simulink model "p1_digital_twin"  (R2023a)
settings: Solver=FixedStepDiscrete  StartTime=0.0  StopTime=10  FixedStep=Ts  RelTol=1e-3  EnableMultiTasking=on
undefined symbols (not defined in the file or in its folder): ack, cpr_handwheel, cpr_steering, DiscIntNeverNeededParam, hal_filter_den, hal_filter_num, n_drive, n_handwheel, n_steering, p1params, param, sr, steering_limit, Ts, wc
libraries: simulink x7
(part 4 of 4)

== system p1_digital_twin/Driver and Controller Input/Steering Controller/HAL-9000/Chirp Signal ==
  note: freqSlope = deltaFreq/targetTime;
      | instantaneousFreq(t) = freqSlope*t + initialFreq;
      | intantaneousPhase(t) = integral(instFreq) = ...
      |       0.5*freqSlope*t^2 + initialFreq*t;
      | outputSignal(t) = sin(instantaneousPhase(t));
  Start Time : Inport
  Digital Clock : DigitalClock  SampleTime=Ts
  Gain : Gain  DisableCoverage=on  Gain=0.5  OutDataTypeStr=Inherit: Same as input  ParamDataTypeStr=Inherit: Same as input
  Output : Trigonometry
  Product : Product  DisableCoverage=on  Inputs=*/  InputSameDT=on  SaturateOnIntegerOverflow=on  OutDataTypeStr=Inherit: Same as first input
  Product1 : Product  DisableCoverage=on  InputSameDT=on  SaturateOnIntegerOverflow=on  OutDataTypeStr=Inherit: Same as first input
  Product2 : Product  DisableCoverage=on  InputSameDT=on  SaturateOnIntegerOverflow=on  OutDataTypeStr=Inherit: Same as first input
  Saturation : Saturate  UpperLimit=duration  LowerLimit=0
  Sum : Sum  DisableCoverage=on  Inputs=|++  InputSameDT=on  SaturateOnIntegerOverflow=on  OutDataTypeStr=Inherit: Same as first input
  Sum1 : Sum  DisableCoverage=on  Inputs=-+|  InputSameDT=on  SaturateOnIntegerOverflow=on  OutDataTypeStr=Inherit: Same as first input
  deltaFreq : Constant  DisableCoverage=on  Value=2*pi*(f2-f1)
  initialFreq : Constant  DisableCoverage=on  Value=2*pi*f1
  targetTime : Constant  DisableCoverage=on  Value=T
  Out2 : Outport
  wires:
  Sum1/1 -> Saturation/1
  Digital Clock/1 -> Sum1/2
  Start Time/1 -> Sum1/1
  deltaFreq/1 -> Product/1
  targetTime/1 -> Product/2
  Product/1 -> Gain/1
  Gain/1 -> Product1/2
  Product1/1 -> Sum/1
  initialFreq/1 -> Sum/2
  Sum/1 -> Product2/2
  Product2/1 -> Output/1
  Output/1 -> Out2/1
  Saturation/1 -> Product1/1, Product2/1

== system p1_digital_twin/Driver and Controller Input/Steering Controller/HAL-9000/Double chirp ==
  In1 : Inport
  Chirp One : Subsystem  mask(chirp){f1=startfreq, T=duration/2, f2=endfreq, VectorParams1D=on}
      mask prompts: f1 "Initial frequency (Hz):"; T "Target time (secs):"; f2 "Frequency at target time (Hz):"; VectorParams1D "Interpret vectors parameters as 1-D"
      mask help: Output a linear chirp signal (sine wave whose frequency varies linearly with time).
      mask init: same as p1_digital_twin/Driver and Controller Input/Steering Controller/HAL-9000/Chirp Signal
      mask Help: The chirp signal has linearly increasing frequency with time.  This block can be used for spectral analysis of nonlinear systems.
      mask Display: plot(t,sin(t.*t))
  Chirp Two : Subsystem  mask(chirp){f1=startfreq, T=duration/2, f2=endfreq, VectorParams1D=on}
      mask prompts: f1 "Initial frequency (Hz):"; T "Target time (secs):"; f2 "Frequency at target time (Hz):"; VectorParams1D "Interpret vectors parameters as 1-D"
      mask help: Output a linear chirp signal (sine wave whose frequency varies linearly with time).
      mask init: same as p1_digital_twin/Driver and Controller Input/Steering Controller/HAL-9000/Chirp Signal
      mask Help: The chirp signal has linearly increasing frequency with time.  This block can be used for spectral analysis of nonlinear systems.
      mask Display: plot(t,sin(t.*t))
  Digital Clock : DigitalClock  SampleTime=Ts
  Relational Operator : RelationalOperator  Operator=<=  OutDataTypeStr=float('double')  InputSameDT=off
  Sum : Sum  DisableCoverage=on  Inputs=++|  InputSameDT=on  SaturateOnIntegerOverflow=on  OutDataTypeStr=Inherit: Same as first input
  Switch : Switch  Threshold=.5  SaturateOnIntegerOverflow=off  InputSameDT=off
  initialFreq : Constant  DisableCoverage=on  Value=duration/2
  Out1 : Outport
  wires:
  Digital Clock/1 -> Relational Operator/1
  Relational Operator/1 -> Switch/2
  initialFreq/1 -> Sum/2
  Sum/1 -> Relational Operator/2, Chirp Two/1(Start Time)
  In1/1 -> Sum/1, Chirp One/1(Start Time)
  Switch/1 -> Out1/1
  Chirp Two/1(Out2) -> Switch/3
  Chirp One/1(Out2) -> Switch/1

== system p1_digital_twin/Driver and Controller Input/Steering Controller/HAL-9000/Double-step ==
  Start Time : Inport
  Data Type Conversion : DataTypeConversion  OutDataTypeStr=double  SaturateOnIntegerOverflow=off  RndMeth=Floor
  Data Type Conversion1 : DataTypeConversion  OutDataTypeStr=double  SaturateOnIntegerOverflow=off  RndMeth=Floor
  Digital Clock : DigitalClock  SampleTime=Ts
  Left Pulse : simulink/Logic and Bit Operations/Interval Test  IntervalClosedRight=off  uplimit=duration  IntervalClosedLeft=on  lowlimit=0  OutDataTypeStr=boolean
  Right Pulse : simulink/Logic and Bit Operations/Interval Test  IntervalClosedRight=off  uplimit=3*duration  IntervalClosedLeft=on  lowlimit=2*duration  OutDataTypeStr=boolean
  Sum : Sum  Inputs=+|-
  Sum1 : Sum  Inputs=+|-
  Out : Outport
  wires:
  Data Type Conversion1/1 -> Sum1/2
  Data Type Conversion/1 -> Sum1/1
  Left Pulse/1 -> Data Type Conversion/1
  Right Pulse/1 -> Data Type Conversion1/1
  Sum1/1 -> Out/1
  Sum/1 -> Right Pulse/1, Left Pulse/1
  Digital Clock/1 -> Sum/1
  Start Time/1 -> Sum/2

== system p1_digital_twin/Driver and Controller Input/Steering Controller/HAL-9000/Latch ==
  In1 : Inport
  Trigger : TriggerPort  VariantControl=(inherit)
  Out1 : Outport
  wires:
  In1/1 -> Out1/1

== system p1_digital_twin/Driver and Controller Input/Steering Controller/HAL-9000/Ramp ==
  Start Time : Inport
  Digital Clock : DigitalClock  SampleTime=Ts
  Saturation : Saturate  UpperLimit=1  LowerLimit=0
  Slope : Gain  Gain=1/duration
  Sum : Sum  DisableCoverage=on  Inputs=|+-  InputSameDT=on  SaturateOnIntegerOverflow=on  OutDataTypeStr=Inherit: Same as first input
  Out1 : Outport
  wires:
  Slope/1 -> Saturation/1
  Saturation/1 -> Out1/1
  Sum/1 -> Slope/1
  Start Time/1 -> Sum/2
  Digital Clock/1 -> Sum/1

== system p1_digital_twin/Driver and Controller Input/Steering Controller/HAL-9000/Step ==
  Start Time : Inport
  Digital Clock : DigitalClock  SampleTime=Ts
  Relational Operator : RelationalOperator  OutDataTypeStr=float('double')  InputSameDT=off
  Out : Outport
  wires:
  Start Time/1 -> Relational Operator/2
  Digital Clock/1 -> Relational Operator/1
  Relational Operator/1 -> Out/1

== system p1_digital_twin/Driver and Controller Input/Steering Controller/HAL-9000/Double chirp/Chirp One ==
  note: freqSlope = deltaFreq/targetTime;
      | instantaneousFreq(t) = freqSlope*t + initialFreq;
      | intantaneousPhase(t) = integral(instFreq) = ...
      |       0.5*freqSlope*t^2 + initialFreq*t;
      | outputSignal(t) = sin(instantaneousPhase(t));
  Start Time : Inport
  Digital Clock : DigitalClock  SampleTime=Ts
  Gain : Gain  DisableCoverage=on  Gain=0.5  OutDataTypeStr=Inherit: Same as input  ParamDataTypeStr=Inherit: Same as input
  Output : Trigonometry
  Product : Product  DisableCoverage=on  Inputs=*/  InputSameDT=on  SaturateOnIntegerOverflow=on  OutDataTypeStr=Inherit: Same as first input
  Product1 : Product  DisableCoverage=on  InputSameDT=on  SaturateOnIntegerOverflow=on  OutDataTypeStr=Inherit: Same as first input
  Product2 : Product  DisableCoverage=on  InputSameDT=on  SaturateOnIntegerOverflow=on  OutDataTypeStr=Inherit: Same as first input
  Saturation : Saturate  UpperLimit=duration/2  LowerLimit=0
  Sum : Sum  DisableCoverage=on  Inputs=|++  InputSameDT=on  SaturateOnIntegerOverflow=on  OutDataTypeStr=Inherit: Same as first input
  Sum1 : Sum  DisableCoverage=on  Inputs=-+|  InputSameDT=on  SaturateOnIntegerOverflow=on  OutDataTypeStr=Inherit: Same as first input
  deltaFreq : Constant  DisableCoverage=on  Value=2*pi*(f2-f1)
  initialFreq : Constant  DisableCoverage=on  Value=2*pi*f1
  targetTime : Constant  DisableCoverage=on  Value=T
  Out2 : Outport
  wires:
  Sum1/1 -> Saturation/1
  Digital Clock/1 -> Sum1/2
  Start Time/1 -> Sum1/1
  deltaFreq/1 -> Product/1
  targetTime/1 -> Product/2
  Product/1 -> Gain/1
  Gain/1 -> Product1/2
  Product1/1 -> Sum/1
  initialFreq/1 -> Sum/2
  Sum/1 -> Product2/2
  Product2/1 -> Output/1
  Output/1 -> Out2/1
  Saturation/1 -> Product1/1, Product2/1

== system p1_digital_twin/Driver and Controller Input/Steering Controller/HAL-9000/Double chirp/Chirp Two ==
  note: freqSlope = deltaFreq/targetTime;
      | instantaneousFreq(t) = freqSlope*t + initialFreq;
      | intantaneousPhase(t) = integral(instFreq) = ...
      |       0.5*freqSlope*t^2 + initialFreq*t;
      | outputSignal(t) = sin(instantaneousPhase(t));
  Start Time : Inport
  Digital Clock : DigitalClock  SampleTime=Ts
  Gain : Gain  DisableCoverage=on  Gain=0.5  OutDataTypeStr=Inherit: Same as input  ParamDataTypeStr=Inherit: Same as input
  Output : Trigonometry
  Product : Product  DisableCoverage=on  Inputs=*/  InputSameDT=on  SaturateOnIntegerOverflow=on  OutDataTypeStr=Inherit: Same as first input
  Product1 : Product  DisableCoverage=on  InputSameDT=on  SaturateOnIntegerOverflow=on  OutDataTypeStr=Inherit: Same as first input
  Product2 : Product  DisableCoverage=on  InputSameDT=on  SaturateOnIntegerOverflow=on  OutDataTypeStr=Inherit: Same as first input
  Saturation : Saturate  UpperLimit=duration/2  LowerLimit=0
  Sum : Sum  DisableCoverage=on  Inputs=|++  InputSameDT=on  SaturateOnIntegerOverflow=on  OutDataTypeStr=Inherit: Same as first input
  Sum1 : Sum  DisableCoverage=on  Inputs=-+|  InputSameDT=on  SaturateOnIntegerOverflow=on  OutDataTypeStr=Inherit: Same as first input
  deltaFreq : Constant  DisableCoverage=on  Value=2*pi*(f2-f1)
  initialFreq : Constant  DisableCoverage=on  Value=2*pi*f1
  targetTime : Constant  DisableCoverage=on  Value=T
  Out2 : Outport
  wires:
  Sum1/1 -> Saturation/1
  Digital Clock/1 -> Sum1/2
  Start Time/1 -> Sum1/1
  deltaFreq/1 -> Product/1
  targetTime/1 -> Product/2
  Product/1 -> Gain/1
  Gain/1 -> Product1/2
  Product1/1 -> Sum/1
  initialFreq/1 -> Sum/2
  Sum/1 -> Product2/2
  Product2/1 -> Output/1
  Output/1 -> Out2/1
  Saturation/1 -> Product1/1, Product2/1
